simulink model "z_control_22b"  (R2022b)
settings: Solver=VariableStepAuto  StartTime=0.0  StopTime=10.0  RelTol=1e-3
InitFcn:
  | init_z_control
undefined symbols (not defined in the file or in its folder): pa
settings Model: Creator=dzxion_microsoft  LastModifiedBy=dzxion_microsoft
settings OptimizationCC: ReuseModelBlockBuffer=on

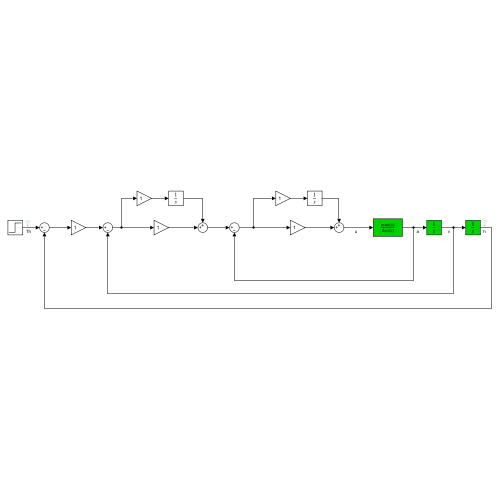
[thumbnail: Simulink's stored preview of the top-level diagram]
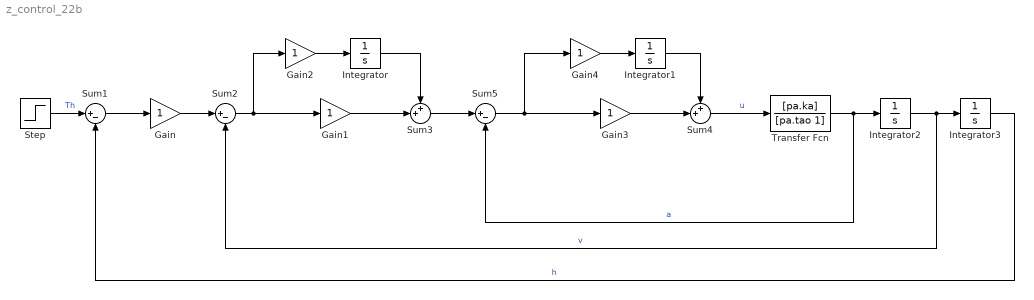
== system z_control_22b ==
  Gain{,1..4} (5 alike) : Gain
  Integrator{,1..3} (4 alike) : Integrator
  Step : Step  SampleTime=0
  Sum1 : Sum  Inputs=|+-
  Sum2 : Sum  Inputs=|+-
  Sum3 : Sum  Inputs=++|
  Sum4 : Sum  Inputs=++|
  Sum5 : Sum  Inputs=|+-
  Transfer Fcn : TransferFcn  Numerator=[pa.ka]  Denominator=[pa.tao 1]
  wires:
  Step/1 -> Sum1/1  "Th"
  Sum1/1 -> Gain/1
  Gain/1 -> Sum2/1
  Sum2/1 -> Gain2/1, Gain1/1
  Gain2/1 -> Integrator/1
  Gain1/1 -> Sum3/2
  Integrator/1 -> Sum3/1
  Gain4/1 -> Integrator1/1
  Integrator1/1 -> Sum4/1
  Gain3/1 -> Sum4/2
  Transfer Fcn/1 -> Sum5/2, Integrator2/1  "a"
  Sum4/1 -> Transfer Fcn/1  "u"
  Integrator2/1 -> Sum2/2, Integrator3/1  "v"
  Integrator3/1 -> Sum1/2  "h"
  Sum3/1 -> Sum5/1
  Sum5/1 -> Gain4/1, Gain3/1
